simulink model "SimLabS"  (R2021a)
settings: Solver=ode3  StartTime=0.0  StopTime=10  FixedStep=0.01  RelTol=1e-3  EnableMultiTasking=on
undefined symbols (not defined in the file or in its folder): Advantech, PCI
libraries: sldrtlib x2
settings Model: SimulationMode=external  ExtModeTrigDuration=20000  ExtModeArchiveFileName=LaboSCL.mat  ExtModeArchiveDirName=Resultats_simul  Creator=erpou15  LastModifiedBy=mabo1165
settings SolverCC: AlgebraicLoopSolver=TrustRegion
settings DataIOCC: MaxDataPoints=15000  SaveFormat=Array  SignalLoggingSaveFormat=ModelDataLogs  SaveOutput=off  SaveTime=off  ReturnWorkspaceOutputs=off
settings OptimizationCC: ExpressionDepthLimit=2147483647  InitFltsAndDblsToZero=on
settings DebuggingCC: ConsistencyChecking=warning  SaveWithParameterizedLinksMsg=none  UnderspecifiedInitializationDetection=Classic  MergeDetectMultiDrivingBlocksExec=none  SignalResolutionControl=TryResolveAllWithWarning  SolverPrmCheckMsg=warning  MultiTaskDSMMsg=warning  MultiTaskCondExecSysMsg=none  FcnCallInpInsideContextMsg=warning  StateNameClashWarn=warning  SFUnexpectedBacktrackingDiag=warning  SFNoUnconditionalDefaultTransitionDiag=warning  SFExecutionAtInitializationDiag=none  SFMachineParentedDataDiag=warning  ArithmeticOperatorsInVariantConditions=warning
settings HardwareCC: TargetHWDeviceType=32-bit Generic
settings ModelReferenceCC: PropagateSignalLabelsOutOfModel=off
settings SFSimCC: SimUseLocalCustomCode=off  CustomCodeUndefinedFunction=UseInterfaceOnly
settings RTWCC: Description=Simulink Desktop Real-Time  SystemTargetFile=sldrt.tlc  TemplateMakefile=sldrt.tmf  RTWUseLocalCustomCode=off  RTWCompilerOptimization=on
settings CodeAppCC: MaxIdLength=95  StateflowObjectComments=on
settings SimulinkDesktopRealTimeCC: TargetPreCompLibLocation=C:\Program Files\MATLAB\R2021a\toolbox\sldrt\lib\win64  TargetLangStandard=C89/C90 (ANSI)  ModelReferenceCompliant=off  CompOptLevelCompliant=off  SupportVariableSizeSignals=off
settings ConfigComp: CovMetricSettings=dw  CovSaveCumulativeToWorkspaceVar=on  CovSaveSingleToWorkspaceVar=on  CovExternalEMLEnable=off  CovSFcnEnable=off

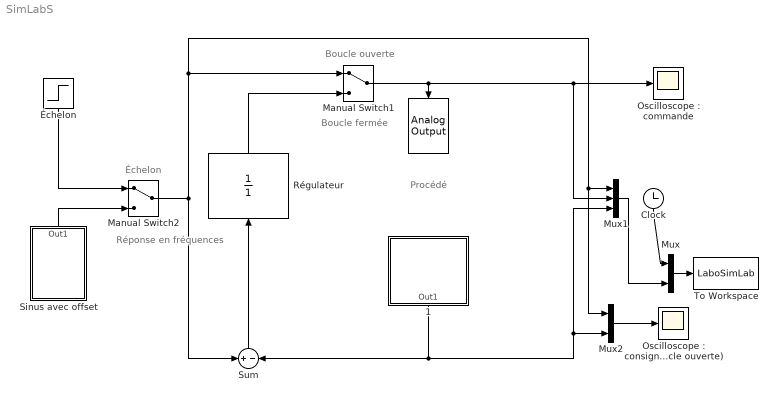
== system SimLabS ==
  note: Boucle ouverte
  note: Boucle fermée
  note: Échelon
  note: Réponse en
      | fréquences
  note: Procédé
  " " : sldrtlib/Analog Output  Tag=Analog output  SampleTime=0  MaxMissedTicks=10  ShowMissedTicks=off  YieldWhenWaiting=off  DrvName=Advantech/PCI-1716  DrvAddress=4294967295  DrvOptions=zeros(1,0)  Channels=1  RangeMode=1  VoltRange=1  InitialValue=0  FinalValue=0
      settings: AttributesFormatString=Advantech\nPCI-1716 [auto]
  " 1" : Subsystem  Tag=Analog Input  mask(Analog Input){InMode=Input 0}
      mask prompts: InMode "Entrée :"
      mask help: Conversion anlogique-numérique.
      mask Help:
      | AUCUNE AIDE DISPONIBLE POUR LE MOMENT
      | VOIR VOTRE GUIDE DE LABORATOIRE
      mask TypeOptions InMode: Input 0 | Input 1
      mask Callback InMode:
      | %if ((strcmp(get_param(gcb, 'InMode'),'Tachymetre (0)')))
      | %	set_param(gcb,'MaskEnables',{'on','on','on','off','on'});
      | %else
      | %    set_param(gcb,'MaskEnables',{'on','off','on','off','on'});
      | %end
      mask Display:
      | port_label('Output',1,'');
      | plot([0 1], [0 0])
      | plot([0 1], [1 1])
      | plot([0 0], [0 1])
      | plot([1 1], [0 1])
      | disp('Analog Input');
  Clock : Clock
      settings: Decimation=1000
  Manual Switch1 : ManualSwitch
  Manual Switch2 : ManualSwitch
  Mux : Mux  Inputs=2
  Mux1 : Mux  Inputs=3
  Mux2 : Mux  Inputs=2
  "Oscilloscope : commande" : Scope
  "Oscilloscope : consigne & sortie (boucle fermée) commande & sortie (boucle ouverte)" : Scope
  Régulateur : TransferFcn  Denominator=[1]
  Sinus avec offset : Subsystem  mask(Sinus avec offset){Amp=0.5, Freq=3.6, Ph=0, Offset=2}
      mask prompts: Amp "Amplitude (V peak) :"; Freq "Fréquence (rad/s) :"; Ph "Phase (rad) :"; Offset "Composante DC (V) :"
      mask help: Générateur de sinusoide avec possibilité d'ajouter une composante DC.
      mask Help:
      | AUCUNE AIDE DISPONIBLE POUR CE BLOC
      | VOIR NOTES DE COURS SCL
      mask Display:
      | port_label('output', 1, '');
      | plot([(0:0.1:(4*pi))+1.5], 1+0.5*sin(0:0.1:(4*pi)));
      | plot([0 4*pi+1.5], [0.25 0.25]);
      | plot([1.5 1.5], [0 2]);
  Sum : Sum  Inputs=+|-  SampleTime=0
  To Workspace : ToWorkspace  VariableName=LaboSimLab  SampleTime=-1
  "Échelon " : Step  SampleTime=0
  wires:
  Manual Switch2/1 -> Manual Switch1/1, Mux1/1, Mux2/1, Sum/1
  Manual Switch1/1 -> Mux1/2, "Oscilloscope : commande"/1, " "/1
  Sum/1 -> Régulateur/1
  Régulateur/1 -> Manual Switch1/2
  Mux2/1 -> "Oscilloscope : consigne & sortie (boucle fermée) commande & sortie (boucle ouverte)"/1
  Mux1/1 -> Mux/2
  "Échelon "/1 -> Manual Switch2/1
  Sinus avec offset/1(Out1) -> Manual Switch2/2
  Mux/1 -> To Workspace/1
  Clock/1 -> Mux/1
  " 1"/1(Out1) -> Sum/2, Mux2/2, Mux1/3

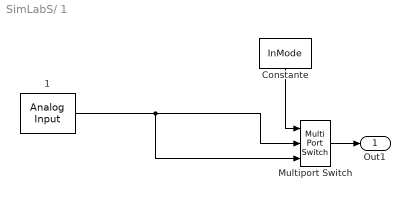
== system SimLabS/ 1 ==
  " 1" : sldrtlib/Analog Input  SampleTime=0  MaxMissedTicks=10  ShowMissedTicks=off  YieldWhenWaiting=off  DrvName=Advantech/PCI-1716  DrvAddress=4294967295  DrvOptions=zeros(1,0)  Channels=InMode  RangeMode=1  VoltRange=2  DataType=1
      settings: AttributesFormatString=Advantech\nPCI-1716 [auto]
  Constante : Constant  Value=InMode
  Multiport Switch : MultiPortSwitch  Inputs=2  RndMeth=Nearest
  Out1 : Outport  VectorParamsAs1DForOutWhenUnconnected=off
  wires:
  Constante/1 -> Multiport Switch/1
  Multiport Switch/1 -> Out1/1
  " 1"/1 -> Multiport Switch/3, Multiport Switch/2

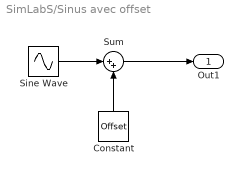
== system SimLabS/Sinus avec offset ==
  Constant : Constant  Value=Offset  SampleTime=0
  Sine Wave : Sin  Amplitude=Amp  Frequency=Freq  Phase=Ph  SampleTime=0
  Sum : Sum  Inputs=|++
  Out1 : Outport  VectorParamsAs1DForOutWhenUnconnected=off
  wires:
  Sine Wave/1 -> Sum/1
  Constant/1 -> Sum/2
  Sum/1 -> Out1/1
